simulink model "PTC_MBDS_StringLeft_Sample"  (R2013a)
settings: Solver=FixedStepDiscrete  StartTime=0.0  StopTime=100  FixedStep=0.02  RelTol=1e-3
undefined symbols (not defined in the file): PTC_MBDS_MaxStringLength_Fcn
libraries: PTC_MBDS_LIB x16, simulink_extras x1
settings Model: Creator=uidl7367  LastModifiedBy=sundeep.tuteja
settings DataIOCC: SignalLoggingSaveFormat=ModelDataLogs
settings OptimizationCC: ExpressionDepthLimit=2147483647  InitFltsAndDblsToZero=on
settings DebuggingCC: SaveWithParameterizedLinksMsg=none  SignalResolutionControl=TryResolveAllWithWarning  SolverPrmCheckMsg=none  InheritedTsInSrcMsg=none  MultiTaskDSMMsg=warning  MultiTaskCondExecSysMsg=none  FcnCallInpInsideContextMsg=UseLocalSettings  StrictBusMsg=Warning
settings RTWCC: IncludeERTFirstTime=on
settings GRTTargetCC: TargetFcnLib=ansi_tfl_tmw.mat  CombineOutputUpdateFcns=off  GRTInterface=on

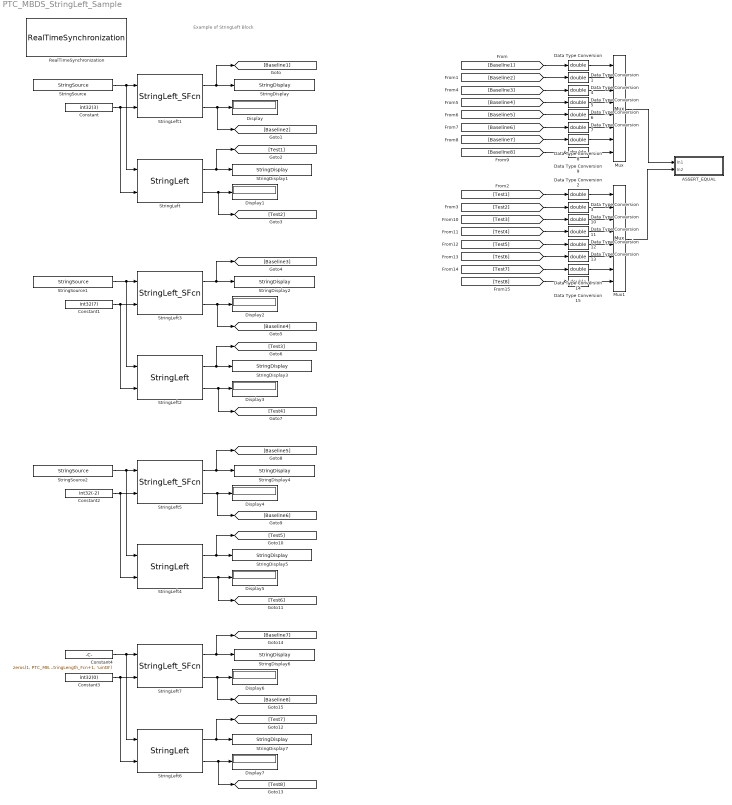
== system PTC_MBDS_StringLeft_Sample ==
  note: Example of StringLeft Block
  ASSERT_EQUAL : Subsystem
  Constant : Constant  InitFcn=|  Value=int32(3)  VectorParams1D=off
      | if(exist('MBDS_BlockCallback', 'file'))
      |    MBDS_BlockCallback('Update', gcb);  
      | end
  Constant1 : Constant  InitFcn=|  Value=int32(7)  VectorParams1D=off
      | if(exist('MBDS_BlockCallback', 'file'))
      |    MBDS_BlockCallback('Update', gcb);  
      | end
  Constant2 : Constant  InitFcn=|  Value=int32(-2)  VectorParams1D=off
      | if(exist('MBDS_BlockCallback', 'file'))
      |    MBDS_BlockCallback('Update', gcb);  
      | end
  Constant3 : Constant  InitFcn=|  Value=int32(0)  VectorParams1D=off
      | if(exist('MBDS_BlockCallback', 'file'))
      |    MBDS_BlockCallback('Update', gcb);  
      | end
  Constant4 : Constant  InitFcn=|  Value=zeros(1, PTC_MBDS_MaxStringLength_Fcn+1, 'uint8')  VectorParams1D=off
      | if(exist('MBDS_BlockCallback', 'file'))
      |    MBDS_BlockCallback('Update', gcb);  
      | end
  Data Type Conversion{,1..15} (16 alike) : DataTypeConversion  OutDataTypeStr=double
  Display{,1..7} (8 alike) : Display
  Mux : Mux  Inputs=8
  Mux1 : Mux  Inputs=8
  RealTimeSynchronization : PTC_MBDS_LIB/MBDS Standard Library/Extended Operations/HMI/RealTimeSynchronization  Enable=off  PTC_MBDS_BlockVersion=5.32  PTC_BlockType=PTC_MBDS_RealTimeSynchronization
  StringDisplay : PTC_MBDS_LIB/MBDS Standard Library/Extended Operations/String Operations/StringDisplay  MaxRowCount=1  BlockSignature=----------  PTC_MBDS_BlockVersion=5.32  PTC_BlockType=PTC_MBDS_StringDisplay  DisplayString=abc  MaxStringLength=PTC_MBDS_MaxStringLength_Fcn
  StringDisplay1 : PTC_MBDS_LIB/MBDS Standard Library/Extended Operations/String Operations/StringDisplay  MaxRowCount=1  BlockSignature=----------  PTC_MBDS_BlockVersion=5.32  PTC_BlockType=PTC_MBDS_StringDisplay  DisplayString=abc  MaxStringLength=PTC_MBDS_MaxStringLength_Fcn
  StringDisplay2 : PTC_MBDS_LIB/MBDS Standard Library/Extended Operations/String Operations/StringDisplay  MaxRowCount=1  BlockSignature=----------  PTC_MBDS_BlockVersion=5.32  PTC_BlockType=PTC_MBDS_StringDisplay  DisplayString=abcde  MaxStringLength=PTC_MBDS_MaxStringLength_Fcn
  StringDisplay3 : PTC_MBDS_LIB/MBDS Standard Library/Extended Operations/String Operations/StringDisplay  MaxRowCount=1  BlockSignature=----------  PTC_MBDS_BlockVersion=5.32  PTC_BlockType=PTC_MBDS_StringDisplay  DisplayString=abcde  MaxStringLength=PTC_MBDS_MaxStringLength_Fcn
  StringDisplay{4..7} (4 alike) : PTC_MBDS_LIB/MBDS Standard Library/Extended Operations/String Operations/StringDisplay  MaxRowCount=1  BlockSignature=----------  PTC_MBDS_BlockVersion=5.32  PTC_BlockType=PTC_MBDS_StringDisplay  MaxStringLength=PTC_MBDS_MaxStringLength_Fcn
  StringLeft{,2,4,6} (4 alike) : PTC_MBDS_LIB/MBDS Standard Library/Extended Operations/String Operations/StringLeft  ENO_Enabled=on  MaxStringLength=PTC_MBDS_MaxStringLength_Fcn  PTC_MBDS_BlockVersion=5.32  PTC_BlockType=PTC_MBDS_StringLeft
  StringLeft1 : S-Function  InitFcn=|  FunctionName=StringLeft_SFcn  Parameters=boolean(ENO_Enabled), uint16(MaxStringLength)  EnableBusSupport=off  mask(StringLeft){MBDS_LibraryBlock=on, ENO_Enabled=on, MBDS_BlockVersion=05.40}
      | if(exist('MBDS_BlockCallback', 'file'))
      |    MBDS_BlockCallback('Update', gcb);
      | end
      mask prompts: MBDS_LibraryBlock "MBDS Library Block"; ENO_Enabled "Show ENO port"; MBDS_BlockVersion "Block version:"
      mask help: The left L characters of the string are extracted. If L is larger then the string length, the result will be the unchanged input and the ENO output is set to false.
      mask init:
      | MBDS_BlockCallback('Copy', gcb);
      | MaxStringLength = 1 + GetStringLen();
      | maskdisplay = 'disp(''Left'')';
      | maskdisplay = sprintf('%s\n%s', maskdisplay, 'port_label(''input'', 1, ''In'')');
      | maskdisplay = sprintf('%s\n%s', maskdisplay, 'port_label(''input'', 2, ''L'')');
      | maskdisplay = sprintf('%s\n%s', maskdisplay, 'port_label(''output'', 1, ''Out'')');
      | if(ENO_Enabled)
      | 	maskdisplay = sprintf('%s\n%s', maskdisplay, 'port_label(''output'', 2, ''ENO'')');
      | end
      | set_param(gcbh, 'maskdisplay', maskdisplay)
      mask Help: eval(['open([workdir(''Library_Dir:''),''\Blockset\Help\'',get_param(gcb,''MaskType''),''.html''])'])
      mask Display:
      | disp('Left')
      | port_label('input', 1, 'In')
      | port_label('input', 2, 'L')
      | port_label('output', 1, 'Out')
      | port_label('output', 2, 'ENO')
  StringLeft3 : S-Function  InitFcn=|  FunctionName=StringLeft_SFcn  Parameters=boolean(ENO_Enabled), uint16(MaxStringLength)  EnableBusSupport=off  mask(StringLeft){MBDS_LibraryBlock=on, ENO_Enabled=on, MBDS_BlockVersion=05.40}
      | if(exist('MBDS_BlockCallback', 'file'))
      |    MBDS_BlockCallback('Update', gcb);
      | end
      mask prompts: MBDS_LibraryBlock "MBDS Library Block"; ENO_Enabled "Show ENO port"; MBDS_BlockVersion "Block version:"
      mask help: The left L characters of the string are extracted. If L is larger then the string length, the result will be the unchanged input and the ENO output is set to false.
      mask init: same as PTC_MBDS_StringLeft_Sample/StringLeft1
      mask Help: eval(['open([workdir(''Library_Dir:''),''\Blockset\Help\'',get_param(gcb,''MaskType''),''.html''])'])
      mask Display:
      | disp('Left')
      | port_label('input', 1, 'In')
      | port_label('input', 2, 'L')
      | port_label('output', 1, 'Out')
      | port_label('output', 2, 'ENO')
  StringLeft5 : S-Function  InitFcn=|  FunctionName=StringLeft_SFcn  Parameters=boolean(ENO_Enabled), uint16(MaxStringLength)  EnableBusSupport=off  mask(StringLeft){MBDS_LibraryBlock=on, ENO_Enabled=on, MBDS_BlockVersion=05.40}
      | if(exist('MBDS_BlockCallback', 'file'))
      |    MBDS_BlockCallback('Update', gcb);
      | end
      mask prompts: MBDS_LibraryBlock "MBDS Library Block"; ENO_Enabled "Show ENO port"; MBDS_BlockVersion "Block version:"
      mask help: The left L characters of the string are extracted. If L is larger then the string length, the result will be the unchanged input and the ENO output is set to false.
      mask init: same as PTC_MBDS_StringLeft_Sample/StringLeft1
      mask Help: eval(['open([workdir(''Library_Dir:''),''\Blockset\Help\'',get_param(gcb,''MaskType''),''.html''])'])
      mask Display:
      | disp('Left')
      | port_label('input', 1, 'In')
      | port_label('input', 2, 'L')
      | port_label('output', 1, 'Out')
      | port_label('output', 2, 'ENO')
  StringLeft7 : S-Function  InitFcn=|  FunctionName=StringLeft_SFcn  Parameters=boolean(ENO_Enabled), uint16(MaxStringLength)  EnableBusSupport=off  mask(StringLeft){MBDS_LibraryBlock=on, ENO_Enabled=on, MBDS_BlockVersion=05.40}
      | if(exist('MBDS_BlockCallback', 'file'))
      |    MBDS_BlockCallback('Update', gcb);
      | end
      mask prompts: MBDS_LibraryBlock "MBDS Library Block"; ENO_Enabled "Show ENO port"; MBDS_BlockVersion "Block version:"
      mask help: The left L characters of the string are extracted. If L is larger then the string length, the result will be the unchanged input and the ENO output is set to false.
      mask init: same as PTC_MBDS_StringLeft_Sample/StringLeft1
      mask Help: eval(['open([workdir(''Library_Dir:''),''\Blockset\Help\'',get_param(gcb,''MaskType''),''.html''])'])
      mask Display:
      | disp('Left')
      | port_label('input', 1, 'In')
      | port_label('input', 2, 'L')
      | port_label('output', 1, 'Out')
      | port_label('output', 2, 'ENO')
  StringSource : PTC_MBDS_LIB/MBDS Standard Library/Extended Operations/String Operations/StringSource  InputValue=abcde  PTC_MBDS_BlockVersion=5.32  PTC_BlockType=PTC_MBDS_StringSource  Value=uint8([97; 98; 99; 100; 101; 0; 0; 0; 0; 0; 0; 0; 0; 0; 0; 0; 0; 0; 0; 0; 0; 0; 0; 0; 0; 0; 0; 0; 0; 0; 0; 0; 0; 0; 0; 0; 0; 0; 0; 0; 0])  MaxStringLength=PTC_MBDS_MaxStringLength_Fcn
  StringSource1 : PTC_MBDS_LIB/MBDS Standard Library/Extended Operations/String Operations/StringSource  InputValue=abcde  PTC_MBDS_BlockVersion=5.32  PTC_BlockType=PTC_MBDS_StringSource  Value=uint8([97; 98; 99; 100; 101; 0; 0; 0; 0; 0; 0; 0; 0; 0; 0; 0; 0; 0; 0; 0; 0; 0; 0; 0; 0; 0; 0; 0; 0; 0; 0; 0; 0; 0; 0; 0; 0; 0; 0; 0; 0])  MaxStringLength=PTC_MBDS_MaxStringLength_Fcn
  StringSource2 : PTC_MBDS_LIB/MBDS Standard Library/Extended Operations/String Operations/StringSource  InputValue=abcde  PTC_MBDS_BlockVersion=5.32  PTC_BlockType=PTC_MBDS_StringSource  Value=uint8([97; 98; 99; 100; 101; 0; 0; 0; 0; 0; 0; 0; 0; 0; 0; 0; 0; 0; 0; 0; 0; 0; 0; 0; 0; 0; 0; 0; 0; 0; 0; 0; 0; 0; 0; 0; 0; 0; 0; 0; 0])  MaxStringLength=PTC_MBDS_MaxStringLength_Fcn
  wires:
  Mux/1 -> ASSERT_EQUAL/1(In1)
  Mux1/1 -> ASSERT_EQUAL/2(In2)
  Data Type Conversion/1 -> Mux/1
  Data Type Conversion1/1 -> Mux/2
  StringSource/1 -> StringLeft1/1, StringLeft/1
  Constant/1 -> StringLeft1/2, StringLeft/2
  StringLeft/2 -> [Test2], Display1/1
  StringLeft1/2 -> [Baseline2], Display/1
  StringLeft/1 -> StringDisplay1/1, [Test1]
  StringLeft1/1 -> StringDisplay/1, [Baseline1]
  [Baseline1] -> Data Type Conversion/1
  [Baseline2] -> Data Type Conversion1/1
  StringSource1/1 -> StringLeft3/1, StringLeft2/1
  Constant1/1 -> StringLeft3/2, StringLeft2/2
  StringLeft2/2 -> [Test4], Display3/1
  StringLeft3/2 -> [Baseline4], Display2/1
  StringLeft2/1 -> StringDisplay3/1, [Test3]
  StringLeft3/1 -> StringDisplay2/1, [Baseline3]
  StringSource2/1 -> StringLeft5/1, StringLeft4/1
  Constant2/1 -> StringLeft5/2, StringLeft4/2
  StringLeft4/2 -> [Test6], Display5/1
  StringLeft5/2 -> [Baseline6], Display4/1
  StringLeft4/1 -> StringDisplay5/1, [Test5]
  StringLeft5/1 -> StringDisplay4/1, [Baseline5]
  Constant4/1 -> StringLeft7/1, StringLeft6/1
  Constant3/1 -> StringLeft7/2, StringLeft6/2
  StringLeft6/2 -> [Test8], Display7/1
  StringLeft7/2 -> [Baseline8], Display6/1
  StringLeft6/1 -> StringDisplay7/1, [Test7]
  StringLeft7/1 -> StringDisplay6/1, [Baseline7]
  Data Type Conversion4/1 -> Mux/3
  Data Type Conversion5/1 -> Mux/4
  [Baseline3] -> Data Type Conversion4/1
  [Baseline4] -> Data Type Conversion5/1
  Data Type Conversion6/1 -> Mux/5
  Data Type Conversion7/1 -> Mux/6
  [Baseline5] -> Data Type Conversion6/1
  [Baseline6] -> Data Type Conversion7/1
  Data Type Conversion8/1 -> Mux/7
  Data Type Conversion9/1 -> Mux/8
  [Baseline7] -> Data Type Conversion8/1
  [Baseline8] -> Data Type Conversion9/1
  Data Type Conversion2/1 -> Mux1/1
  Data Type Conversion3/1 -> Mux1/2
  [Test1] -> Data Type Conversion2/1
  [Test2] -> Data Type Conversion3/1
  Data Type Conversion10/1 -> Mux1/3
  Data Type Conversion11/1 -> Mux1/4
  [Test3] -> Data Type Conversion10/1
  [Test4] -> Data Type Conversion11/1
  Data Type Conversion12/1 -> Mux1/5
  Data Type Conversion13/1 -> Mux1/6
  [Test5] -> Data Type Conversion12/1
  [Test6] -> Data Type Conversion13/1
  Data Type Conversion14/1 -> Mux1/7
  Data Type Conversion15/1 -> Mux1/8
  [Test7] -> Data Type Conversion14/1
  [Test8] -> Data Type Conversion15/1

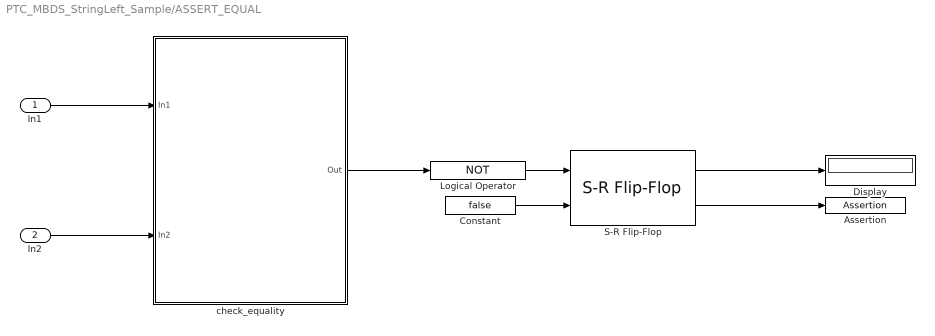
== system PTC_MBDS_StringLeft_Sample/ASSERT_EQUAL ==
  In1 : Inport
  In2 : Inport  Port=2
  Assertion : Assertion
  Constant : Constant  Value=false
  Display : Display
  Logical Operator : Logic  Operator=NOT  AllPortsSameDT=off  OutDataTypeStr=boolean
  S-R Flip-Flop : simulink_extras/Flip Flops/S-R Flip-Flop  initial_condition=0
  check_equality : MATLAB Function  TreatAsAtomicUnit=on
  wires:
  S-R Flip-Flop/1 -> Display/1
  check_equality/1(Out) -> Logical Operator/1
  Constant/1 -> S-R Flip-Flop/2
  S-R Flip-Flop/2 -> Assertion/1
  In2/1 -> check_equality/2(In2)
  In1/1 -> check_equality/1(In1)
  Logical Operator/1 -> S-R Flip-Flop/1

== matlab function PTC_MBDS_StringLeft_Sample/ASSERT_EQUAL/check_equality ==
  data: In1 input; Out output; In2 input
function Out = check_equality(In1, In2)
%#codegen

Out = isequaln(In1, In2);

end
